simulink model "TesteIdentificaoRecursiva"  (R2017b)
settings: Solver=VariableStepAuto  StartTime=0.0  StopTime=14702  RelTol=1e-3
libraries: slident x2
settings Model: Creator=heyderaraujo  LastModifiedBy=heyderaraujo

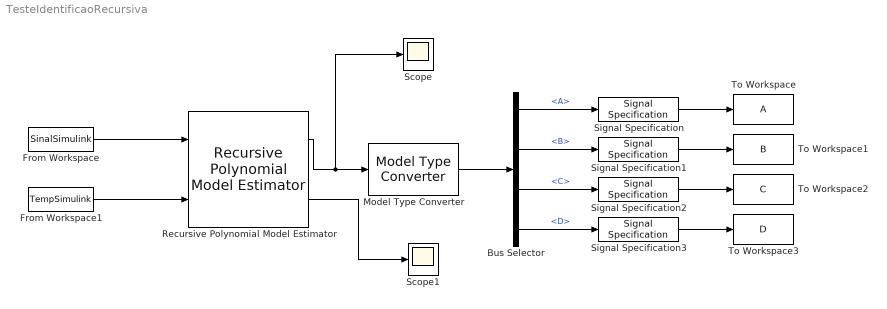
== system TesteIdentificaoRecursiva ==
  Bus Selector : BusSelector  OutputSignals=A,B,C,D
  From Workspace : FromWorkspace  VariableName=SinalSimulink  SampleTime=1
  From Workspace1 : FromWorkspace  VariableName=TempSimulink  SampleTime=1
  Model Type Converter : slident/Estimators/Model Type Converter  InputModelType=ARX
      settings: SourceProductName=System Identification Toolbox  SourceProductBaseCode=ID
  Recursive Polynomial Model Estimator : slident/Estimators/Recursive Polynomial Model Estimator  ModelStructure=ARX  InitialEstimateSource=None  A0=2  B0=1  C0=1  D0=1  F0=1  nk=1  P0=1e4  EstimationMethod=Forgetting Factor  AdaptationParameter=0.956  HasTimeVaryingAdaptationParameter=off  NormalizationBias=eps  OutputError=on  OutputP=off  AddEnablePort=off  Ts=-1
      settings: SourceProductName=System Identification Toolbox  SourceProductBaseCode=ID
  Scope : Scope
  Scope1 : Scope
  Signal Specification : SignalSpecification  Dimensions=[2 2]
  Signal Specification1 : SignalSpecification  Dimensions=[2 1]
  Signal Specification2 : SignalSpecification  Dimensions=[1 2]
  Signal Specification3 : SignalSpecification  Dimensions=[1 1]
  To Workspace : ToWorkspace  VariableName=A  SaveFormat=Timeseries  SampleTime=-1
  To Workspace1 : ToWorkspace  VariableName=B  SaveFormat=Timeseries  SampleTime=-1
  To Workspace2 : ToWorkspace  VariableName=C  SaveFormat=Timeseries  SampleTime=-1
  To Workspace3 : ToWorkspace  VariableName=D  SaveFormat=Timeseries  SampleTime=-1
  wires:
  Recursive Polynomial Model Estimator/1 -> Scope/1, Model Type Converter/1
  Model Type Converter/1 -> Bus Selector/1
  From Workspace/1 -> Recursive Polynomial Model Estimator/1
  From Workspace1/1 -> Recursive Polynomial Model Estimator/2
  Bus Selector/1 -> Signal Specification/1  "<A>"
  Bus Selector/2 -> Signal Specification1/1  "<B>"
  Bus Selector/3 -> Signal Specification2/1  "<C>"
  Bus Selector/4 -> Signal Specification3/1  "<D>"
  Signal Specification/1 -> To Workspace/1
  Signal Specification1/1 -> To Workspace1/1
  Signal Specification2/1 -> To Workspace2/1
  Signal Specification3/1 -> To Workspace3/1
  Recursive Polynomial Model Estimator/2 -> Scope1/1
